simulink model "unicycle_bpoint_posture_reg"  (R2023b)
settings: Solver=ode45  StartTime=0.0  StopTime=30  MaxStep=0.01  MinStep=1e-3  RelTol=1e-3
values from neighbouring files (symbols this model uses):
  initial_condition = [12 0 pi/2]    [init_bpoint.m]    (also in initialize.m)
  parking_spot = [12, -2, pi/2]    [init_bpoint.m]    (also in initialize.m)
  use_posture_regulator = 0    [init_bpoint.m]    (also in initialize.m = 1)
libraries: dspsigops x1
settings Model: Creator=tubaldotom  LastModifiedBy=utente
settings DataIOCC: ReturnWorkspaceOutputs=off
settings OptimizationCC: ReuseModelBlockBuffer=off

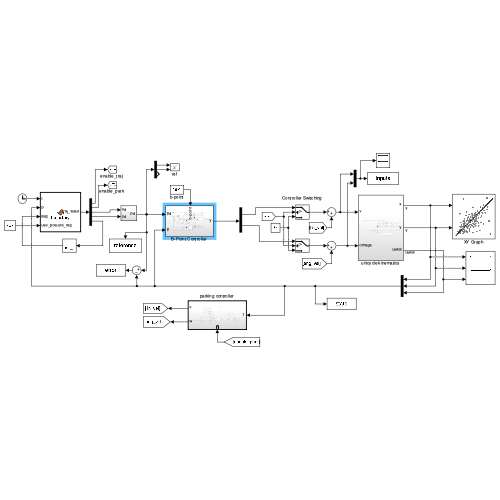
[thumbnail: Simulink's stored preview of the top-level diagram]
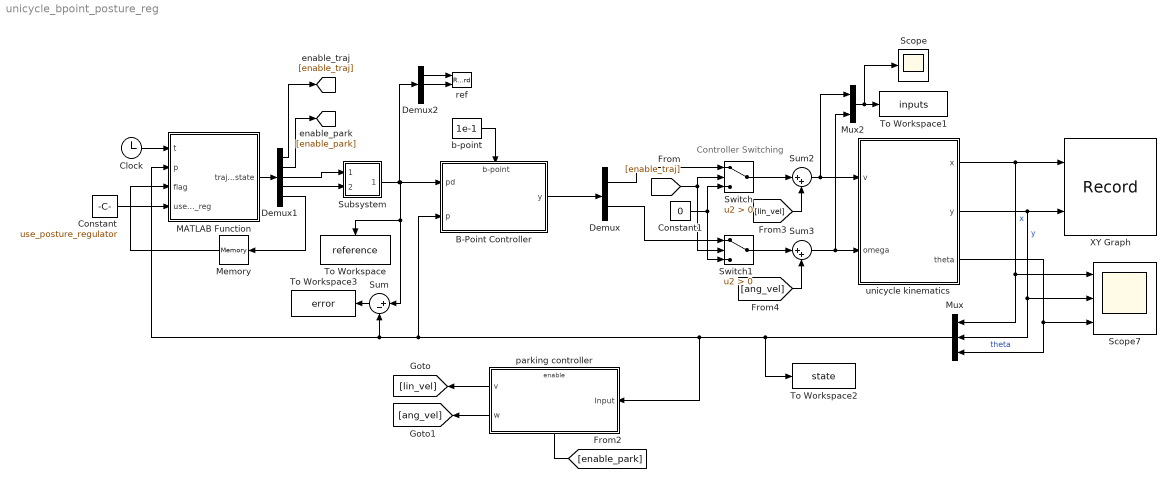
== system unicycle_bpoint_posture_reg ==
  note: Controller Switching
  B-Point Controller : Subsystem
      settings: PortSchema="{\"entries\":[{\"content\":{\"sides\":[{\"content\":{\"connectorIds\":[\"In1\",\"In2\"]},\"type\":\"ConnectorPlacement.EquallySpacedRectSide\",\"uuid\":\"7174ddc3-0332-4984-af4b-f4adb17160f2\"},{\"content\":{\"connectorIds\":[\"Out1\"],\"side\":\"RIGHT\"},\"type\":\"ConnectorPlacement.EquallySpacedRectSide\",\"uuid\":\"ff5d30be-5b89-48b1-a652-8bbfe73cad42\"},{\"content\":{\"connectorIds\":[\"In3\"],\"side\":\"TOP\"},\"type\":\"ConnectorPlacement.EquallySpacedRectSide\",\"uuid\":\"5ae40dfe-ce50-4342-82aa-488d6fa8be95\"}]},\"type\":\"ConnectorPlacement.EquallySpacedConnector\",\"uuid\":\"87d0a50d-c056-438b-b4e5-2fc1827c7218\"}],\"packageUris\":[\"http://schema.mathworks.com/mf0/Connector/R2020b\"],\"version\":\"1.0\"}"
  Clock : Clock
  Constant : Constant  Value=use_posture_regulator
  Constant1 : Constant  Value=0
  Demux : Demux  Outputs=2
  Demux1 : Demux  Outputs=5
  Demux2 : Demux  Outputs=3
  MATLAB Function : MATLAB Function  TreatAsAtomicUnit=on
  Memory : Memory  InitialCondition=1
  Mux : Mux  Inputs=3
  Mux2 : Mux  Inputs=2
  Scope : Scope
  Scope7 : Scope  NumInputPorts=3
  Subsystem : Subsystem
  Sum : Sum  Inputs=|+-
  Sum2 : Sum  Inputs=|++
  Sum3 : Sum  Inputs=|++
  Switch : Switch  Criteria=u2 > Threshold  SaturateOnIntegerOverflow=off  InputSameDT=off
  Switch1 : Switch  Criteria=u2 > Threshold  SaturateOnIntegerOverflow=off  InputSameDT=off
  To Workspace : ToWorkspace  VariableName=reference  SaveFormat=Structure With Time  SampleTime=-1
  To Workspace1 : ToWorkspace  VariableName=inputs  SaveFormat=Structure With Time  SampleTime=-1
  To Workspace2 : ToWorkspace  VariableName=state  SaveFormat=Structure With Time  SampleTime=-1
  To Workspace3 : ToWorkspace  VariableName=error  SaveFormat=Structure With Time  SampleTime=-1
  XY Graph : Record  FileSettingsInternal="{\"entries\":[{\"content\":{\"excelSettings\":{\"content\":{},\"type\":\"Streamout.ExcelSettings\"}},\"type\":\"Streamout.FileSettingStorage\",\"uuid\":\"\"}],\"packageUris\":[\"http:\\/\\/schema.mathworks.com\\/mf0\\/streamout_blocks\\/R2020a\"],\"version\":\"1.0\"}"  Layout=[1 1]  SignalsInternal="{\"entries\":[{\"content\":{\"signals\":[{\"content\":{\"blockPath\":[],\"dimensions\":[1,1],\"domain\":\"\",\"lineColor\":\"#a2142f\",\"plots\":[ 1 ],\"port\":1,\"signalID\":1,\"signalName\":\"x\"},\"type\":\"RecordBlkView.Signal\",\"uuid\":\"\"},{\"content\":{\"blockPath\":[],\"dimensions\":[1,1],\"domain\":\"\",\"lineColor\":\"#139fff\",\"plots\":[ 1 ],\"port\":2,\"signalID\":2,\"signalName\":\"y\"},\"type\":\"RecordBlkView.Signal\",\"uuid\":\"\"}]},\"type\":\"RecordBlkView.InputSignals\",\"uuid\":\"\"}],\"packageUris\":[\"http:\\/\\/schema.mathworks.com\\/mf0\\/streamout_blocks\\/R2020a\"],\"version\":\"1.0\"}"  VisualizationBindings="{\"xyplotplugin\":{\"info\":[{\"series\":[{\"bindingParametersList\":[{\"parameter\":\"X-Axis\",\"signalID\":1,\"signalName\":\"x\"},{\"parameter\":\"Y-Axis\",\"signalID\":2,\"signalName\":\"y\"}],\"seriesID\":0}],\"subplotID\":1}]}}"  CompatibilityTag=XY
  b-point : Constant  Value=1e-1
  parking controller : Subsystem
  ref : Record  FileSettingsInternal="{\"entries\":[{\"content\":{\"excelSettings\":{\"content\":{},\"type\":\"Streamout.ExcelSettings\"}},\"type\":\"Streamout.FileSettingStorage\",\"uuid\":\"\"}],\"packageUris\":[\"http:\\/\\/schema.mathworks.com\\/mf0\\/streamout_blocks\\/R2020a\"],\"version\":\"1.0\"}"  Layout=[1 1]  SignalsInternal="{\"entries\":[{\"content\":{\"signals\":[{\"content\":{\"blockPath\":[],\"dimensions\":[1],\"domain\":\"\",\"lineColor\":\"#a2142f\",\"plots\":[ 1 ],\"port\":1,\"signalID\":1,\"signalName\":\"Demux2:1\"},\"type\":\"RecordBlkView.Signal\",\"uuid\":\"\"},{\"content\":{\"blockPath\":[],\"dimensions\":[1],\"domain\":\"\",\"lineColor\":\"#139fff\",\"plots\":[ 1 ],\"port\":2,\"signalID\":2,\"signalName\":\"Demux2:2\"},\"type\":\"RecordBlkView.Signal\",\"uuid\":\"\"}]},\"type\":\"RecordBlkView.InputSignals\",\"uuid\":\"\"}],\"packageUris\":[\"http:\\/\\/schema.mathworks.com\\/mf0\\/streamout_blocks\\/R2020a\"],\"version\":\"1.0\"}"  VisualizationBindings="{\"xyplotplugin\":{\"info\":[{\"series\":[{\"bindingParametersList\":[{\"parameter\":\"X-Axis\",\"signalID\":1,\"signalName\":\"Demux2:1\"},{\"parameter\":\"Y-Axis\",\"signalID\":2,\"signalName\":\"Demux2:2\"}],\"seriesID\":0}],\"subplotID\":1}]}}"  CompatibilityTag=XY
  unicycle kinematics : Subsystem
  wires:
  unicycle kinematics/1(x) -> XY Graph/1, Scope7/1, Mux/1  "x"
  unicycle kinematics/2(y) -> XY Graph/2, Scope7/2, Mux/2  "y"
  unicycle kinematics/3(theta) -> Scope7/3, Mux/3  "theta"
  Demux1/5 -> Memory/1
  Memory/1 -> MATLAB Function/3(flag)
  Demux1/1 -> [enable_traj]
  Demux1/2 -> [enable_park]
  parking controller/2(w) -> [ang_vel]
  parking controller/1(v) -> [lin_vel]
  [lin_vel] -> Sum2/2
  Constant1/1 -> Switch1/3, Switch/3
  [enable_traj] -> Switch/2, Switch1/2
  [ang_vel] -> Sum3/2
  Demux/1 -> Switch/1
  Demux/2 -> Switch1/1
  Switch/1 -> Sum2/1
  Switch1/1 -> Sum3/1
  Demux1/3 -> Subsystem/1(xd)
  Demux1/4 -> Subsystem/2(yd)
  B-Point Controller/1(y) -> Demux/1
  b-point/1 -> B-Point Controller/3(b-point)
  MATLAB Function/1(traj_state) -> Demux1/1
  Clock/1 -> MATLAB Function/1(t)
  Subsystem/1(pd) -> Demux2/1, Sum/1, To Workspace/1, B-Point Controller/1(pd)
  Mux2/1 -> Scope/1, To Workspace1/1
  Sum3/1 -> Mux2/2, unicycle kinematics/2(omega)
  Sum2/1 -> Mux2/1, unicycle kinematics/1(v)
  Mux/1 -> To Workspace2/1, parking controller/1(Input), MATLAB Function/2(p), Sum/2, B-Point Controller/2(p)
  [enable_park] -> parking controller/Enable
  Constant/1 -> MATLAB Function/4(use_posture_reg)
  Sum/1 -> To Workspace3/1
  Demux2/1 -> ref/1
  Demux2/2 -> ref/2

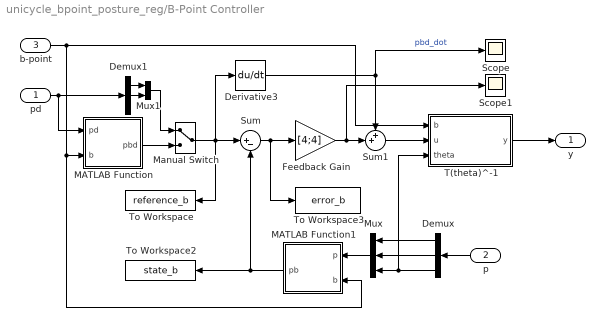
== system unicycle_bpoint_posture_reg/B-Point Controller ==
  pd : Inport
  p : Inport  Port=2
  b-point : Inport  Port=3
  Demux : Demux  Outputs=3
  Demux1 : Demux  Outputs=3
  Derivative3 : Derivative
  Feedback Gain : Gain  Gain=[4;4]
  MATLAB Function : MATLAB Function  TreatAsAtomicUnit=on
  MATLAB Function1 : MATLAB Function  TreatAsAtomicUnit=on
  Manual Switch : ManualSwitch
  Mux : Mux  Inputs=3
  Mux1 : Mux  Inputs=2
  Scope : Scope
  Scope1 : Scope
  Sum : Sum  Inputs=|+-
  Sum1 : Sum  Inputs=++|
  T(theta)^-1 : MATLAB Function  TreatAsAtomicUnit=on
  To Workspace : ToWorkspace  VariableName=reference_b  SaveFormat=Structure With Time  SampleTime=-1
  To Workspace2 : ToWorkspace  VariableName=state_b  SaveFormat=Structure With Time  SampleTime=-1
  To Workspace3 : ToWorkspace  VariableName=error_b  SaveFormat=Structure With Time  SampleTime=-1
  y : Outport
  wires:
  MATLAB Function1/1(pb) -> Sum/2, To Workspace2/1
  Derivative3/1 -> Scope/1, Sum1/1  "pbd_dot"
  Sum1/1 -> T(theta)^-1/2(u)
  Demux/3 -> T(theta)^-1/3(theta), Mux/3
  Feedback Gain/1 -> Scope1/1, Sum1/2
  Sum/1 -> To Workspace3/1, Feedback Gain/1
  p/1 -> Demux/1
  Mux/1 -> MATLAB Function1/1(p)
  Demux/1 -> Mux/1
  Demux/2 -> Mux/2
  b-point/1 -> T(theta)^-1/1(b), MATLAB Function1/2(b), MATLAB Function/2(b)
  T(theta)^-1/1(y) -> y/1
  pd/1 -> MATLAB Function/1(pd), Demux1/1
  MATLAB Function/1(pbd) -> Manual Switch/2
  Manual Switch/1 -> Derivative3/1, To Workspace/1, Sum/1
  Demux1/1 -> Mux1/1
  Demux1/2 -> Mux1/2
  Mux1/1 -> Manual Switch/1

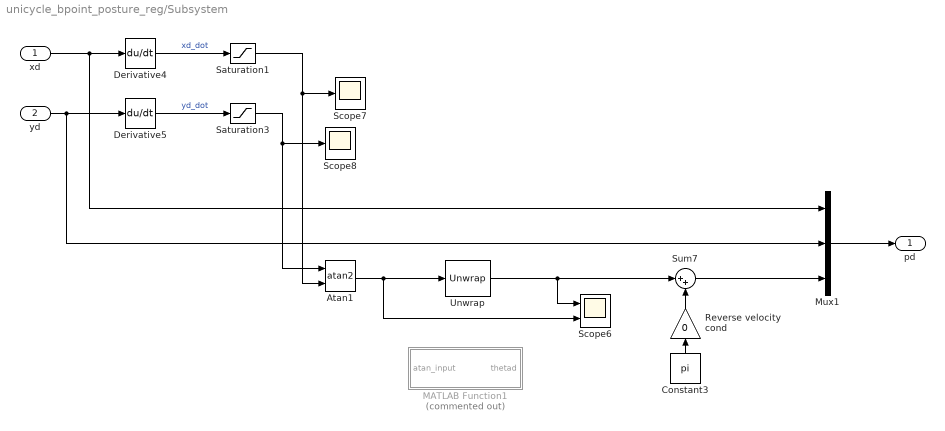
== system unicycle_bpoint_posture_reg/Subsystem ==
  xd : Inport
  yd : Inport  Port=2
  Atan1 : Trigonometry  Operator=atan2
  Constant3 : Constant  Value=pi
  Derivative4 : Derivative
  Derivative5 : Derivative
  MATLAB Function1 : MATLAB Function  Commented=on  TreatAsAtomicUnit=on
  Mux1 : Mux  Inputs=3
  Reverse velocity cond : Gain  Gain=0
  Saturation1 : Saturate  UpperLimit=100  LowerLimit=-100  ZeroCross=off
  Saturation3 : Saturate  UpperLimit=100  LowerLimit=-100  ZeroCross=off
  Scope6 : Scope  NumInputPorts=2
  Scope7 : Scope
  Scope8 : Scope
  Sum7 : Sum  Inputs=|++
  Unwrap : dspsigops/Unwrap  tol=pi  InputProcessing=Columns as channels (frame based)  running=off
  pd : Outport
  wires:
  Sum7/1 -> Mux1/3
  Derivative5/1 -> Saturation3/1  "yd_dot"
  Derivative4/1 -> Saturation1/1  "xd_dot"
  xd/1 -> Derivative4/1, Mux1/1
  Constant3/1 -> Reverse velocity cond/1
  Reverse velocity cond/1 -> Sum7/2
  yd/1 -> Derivative5/1, Mux1/2
  Atan1/1 -> Unwrap/1, Scope6/2
  Mux1/1 -> pd/1
  Saturation3/1 -> Scope8/1, Atan1/1
  Saturation1/1 -> Scope7/1, Atan1/2
  Unwrap/1 -> Scope6/1, Sum7/1

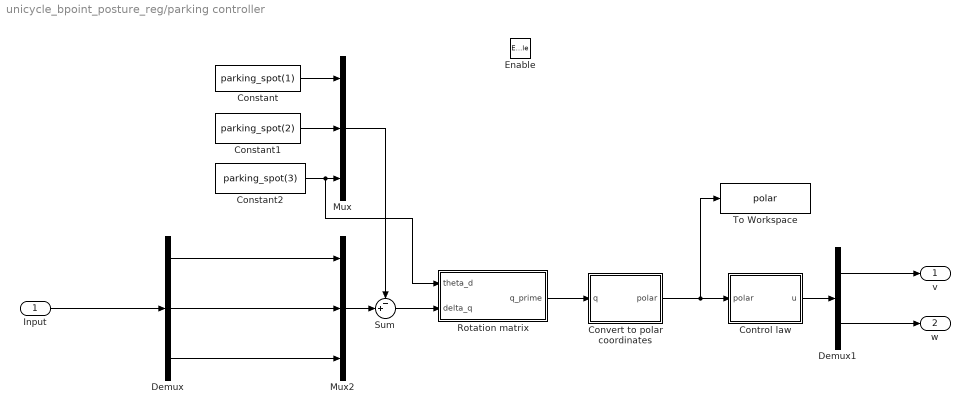
== system unicycle_bpoint_posture_reg/parking controller ==
  Input : Inport
  Enable : EnablePort  StatesWhenEnabling=reset
  Constant : Constant  Value=parking_spot(1)
  Constant1 : Constant  Value=parking_spot(2)
  Constant2 : Constant  Value=parking_spot(3)
  Control law : MATLAB Function  TreatAsAtomicUnit=on
  Convert to polar coordinates : MATLAB Function  TreatAsAtomicUnit=on
  Demux : Demux  Outputs=3
  Demux1 : Demux  Outputs=2
  Mux : Mux  Inputs=3
  Mux2 : Mux  Inputs=3
  Rotation matrix : MATLAB Function  TreatAsAtomicUnit=on
  Sum : Sum  Inputs=-+|
  To Workspace : ToWorkspace  VariableName=polar  SaveFormat=Structure With Time  SampleTime=-1
  v : Outport
  w : Outport  Port=2
  wires:
  Rotation matrix/1(q_prime) -> Convert to polar coordinates/1(q)
  Demux1/2 -> w/1
  Constant2/1 -> Rotation matrix/1(theta_d), Mux/3
  Constant1/1 -> Mux/2
  Mux2/1 -> Sum/2
  Mux/1 -> Sum/1
  Sum/1 -> Rotation matrix/2(delta_q)
  Demux1/1 -> v/1
  Convert to polar coordinates/1(polar) -> Control law/1(polar), To Workspace/1
  Constant/1 -> Mux/1
  Control law/1(u) -> Demux1/1
  Input/1 -> Demux/1
  Demux/2 -> Mux2/2
  Demux/1 -> Mux2/1
  Demux/3 -> Mux2/3

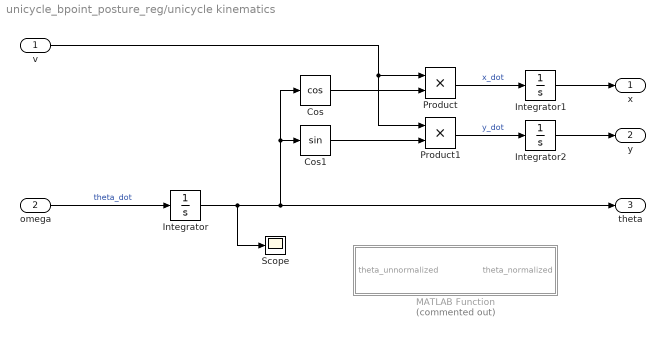
== system unicycle_bpoint_posture_reg/unicycle kinematics ==
  v : Inport
  omega : Inport  Port=2
  Cos : Trigonometry  Operator=cos
  Cos1 : Trigonometry
  Integrator : Integrator  InitialCondition=initial_condition(3)  ZeroCross=off
  Integrator1 : Integrator  InitialCondition=initial_condition(1)
  Integrator2 : Integrator  InitialCondition=initial_condition(2)
  MATLAB Function : MATLAB Function  Commented=on  TreatAsAtomicUnit=on
  Product : Product
  Product1 : Product
  Scope : Scope
  x : Outport
  y : Outport  Port=2
  theta : Outport  Port=3
  wires:
  Integrator/1 -> Scope/1, theta/1, Cos/1, Cos1/1
  Integrator2/1 -> y/1
  Cos1/1 -> Product1/2
  v/1 -> Product/1, Product1/1
  Product1/1 -> Integrator2/1  "y_dot"
  omega/1 -> Integrator/1  "theta_dot"
  Integrator1/1 -> x/1
  Cos/1 -> Product/2
  Product/1 -> Integrator1/1  "x_dot"

== matlab function unicycle_bpoint_posture_reg/B-Point Controller/MATLAB Function ==
  data: pd input; pbd output; b input
function pbd = p2b(pd,b)
pbd = zeros(2,1);
pbd(1) = pd(1) + b*cos(pd(3)); 
pbd(2) = pd(2) + b*sin(pd(3));

== matlab function unicycle_bpoint_posture_reg/MATLAB Function ==
  data: t input; traj_state output; p input; flag input; use_posture_reg input
function traj_state= trajectory(t,p,flag,use_posture_reg)
r1 = 10; % trajectory radius
r2 = 1;  % obstacle avoidance trajectory radius
omega = 0.3;
traj_state = zeros(5,1);

enable_traj = 0;
enable_park = 0;
x = 0;
y = 0;

% a quarter of circle
if(flag == 1)
    enable_traj = 1;
    enable_park = 0;
    x = r1*cos(omega*t);
    y = r1*sin(omega*t);
end

delta_r = 1e-2;   % added to the radius of the obst. avoid. traj. in order to anticipate the switch
if(abs(p(1)) < (1 + delta_r) && abs(p(2) - r1) < (1 + delta_r) && flag==1)
    enable_traj = 1;
    enable_park = 0;
    flag = 2;
end

%obstacle avoidance
if(flag==2)
    enable_traj = 1;
    enable_park = 0;
    x = r2*cos(omega*(t-4.892));   % 4.8924
    y = r1 + r2*sin(omega*(t-4.892));
end

% switch back to traj tracking
if(abs(p(1) + r2)<0.1 && abs(p(2) - r1)<0.1 && flag==2)
    enable_traj = 0;
    enable_park = 1;
    flag = 3;
end

%3/4 of a circle
if(flag==3)
    enable_traj = 1;
    enable_park = 0;
    x = r1*cos(omega*(t - 15.361) + 1.67);  % phase = pi/2 + arcsin(r2/r1)
    y = r1*sin(omega*(t - 15.361) + 1.67);   % 15.034 / 15.075
end

thresh = 1e-1;  % distance from starting point at which the parking procedure starts
if(t>10 && abs(p(1)-r1)<thresh && abs(p(2))<thresh && flag==3)
    if(use_posture_reg==1)
        flag = 4;
        enable_traj = 0;
        enable_park = 1;
    else
        flag = 5;
    end
end

if(flag==4)
    enable_traj = 0;
    enable_park = 1;
end

if(flag==5)
    enable_traj = 0;
    enable_park = 0;
end

flag_out= flag;

traj_state = [enable_traj;enable_park;x;y;flag_out];

== matlab function unicycle_bpoint_posture_reg/unicycle kinematics/MATLAB Function ==
  data: theta_unnormalized input; theta_normalized output
function theta_normalized = normalize_theta(theta_unnormalized)

    theta_normalized = mod(theta_unnormalized, 2*pi);

== matlab function unicycle_bpoint_posture_reg/B-Point Controller/MATLAB Function1 ==
  data: p input; pb output; b input
function pb = p2b(p,b)
pb = zeros(2,1);
pb(1) = p(1) + b*cos(p(3)); 
pb(2) = p(2) + b*sin(p(3));

== matlab function unicycle_bpoint_posture_reg/B-Point Controller/T(theta)^-1 ==
  data: b input; u input; y output; theta input
function y = in_out(b,u,theta)
b = 0.1;
y = zeros(2,1);
T_inv = (1/b)*[b*cos(theta) b*sin(theta); -sin(theta) cos(theta)];
y = T_inv*u;

== matlab function unicycle_bpoint_posture_reg/parking controller/Control law ==
  data: polar input; u output
function u = fcn(polar)
u = zeros(2,1);

rho = polar(1);
gamma = polar(2);
delta = polar(3);

k1 = 3;
k2 = 3;
k3 = 3;

v = k1*rho*cos(gamma);

if ((gamma > 0.01 || gamma < -0.01) || rho > 0.01 || (delta > 0.01 || delta < -0.01))
    w = k2*gamma+(k1*sin(gamma)*cos(gamma)/gamma*(gamma+k3*delta));
else
    w = 0;
    v = 0;
end
u = [v;w];

== matlab function unicycle_bpoint_posture_reg/parking controller/Convert to polar coordinates ==
  data: q input; polar output
function polar = fcn(q)
polar = zeros(3,1);

rho = sqrt(q(1)^2+q(2)^2);
gamma = atan2(q(2),q(1)) + pi - q(3);
delta = gamma + q(3);

polar = [rho; wrapToPi(gamma); wrapToPi(delta)];

% I need to wrap between [-pi, +pi] so that when we are stabilizing
% around 0 we do not continuously switch between 0 and 2pi.
% Here I must not unwrap the angles because the angles are used as 
% multipliers in the computation of w, so they need to be expressed in
% normalized radians.

== matlab function unicycle_bpoint_posture_reg/parking controller/Rotation matrix ==
  data: theta_d input; delta_q input; q_prime output
% I need to express polar coordinates with respect to a rotated frame.
% The rotated frame is obtained by rotating about the z axis of the 
% original one by theta_d radians. 
% So, to express delta_q in that rotated frame I need to change the basis 
% from the original one to the rotated one, and so I multiply delta_q by 
% the inverted (= transposed) rotation matrix.
function q_prime = fcn(theta_d,delta_q)
c = cos(theta_d);
s = sin(theta_d);

% Rotation matrix
R = [c  s   0;
     -s c   0;
     0  0   1];

q_prime = R*delta_q;

== matlab function unicycle_bpoint_posture_reg/Subsystem/MATLAB Function1 ==
  data: atan_input input; thetad output
function thetad = convert_angle(atan_input)
    if(atan_input < 0)
        thetad = atan_input + 2*pi;
    else
        thetad = atan_input;
    end
